simulink model "exintercol"  (R2018a)
settings: Solver=FixedStepDiscrete  StartTime=0.0  StopTime=500  RelTol=1e-3  EnableMultiTasking=on
values from neighbouring files (symbols this model uses):
  lt = 3    [examplesupplychainCIO.m]
undefined symbols (not defined in the file or in its folder): magnitude, norminv
settings Model: Creator=Juan Ramón Trapero  LastModifiedBy=azken
settings DataIOCC: LimitDataPoints=on  SaveFormat=Array  SignalLoggingSaveFormat=ModelDataLogs
settings OptimizationCC: ExpressionDepthLimit=2147483647  InitFltsAndDblsToZero=on  LifeSpan=inf
settings DebuggingCC: UnderspecifiedInitializationDetection=Classic  MergeDetectMultiDrivingBlocksExec=none  SolverPrmCheckMsg=warning  FcnCallInpInsideContextMsg=warning  StateNameClashWarn=warning  SFUnexpectedBacktrackingDiag=warning  SFNoUnconditionalDefaultTransitionDiag=warning  SFExecutionAtInitializationDiag=none
settings HardwareCC: ProdBitPerPointer=32  ProdBitPerSizeT=32  ProdBitPerPtrDiffT=32  ProdLargestAtomicFloat=None  ProdIntDivRoundTo=Undefined  ProdEndianess=Unspecified  ProdWordSize=32  ProdHWDeviceType=32-bit Generic
settings ModelReferenceCC: PropagateSignalLabelsOutOfModel=off
settings CodeAppCC: StateflowObjectComments=on
settings GRTTargetCC: TargetLangStandard=C89/C90 (ANSI)  GeneratePreprocessorConditionals=Disable all  CombineOutputUpdateFcns=off  GRTInterface=on
settings ConfigComp: CovMetricSettings=dw  CovHtmlReporting=on  CovSaveCumulativeToWorkspaceVar=on  CovSaveSingleToWorkspaceVar=on  CovExternalEMLEnable=off

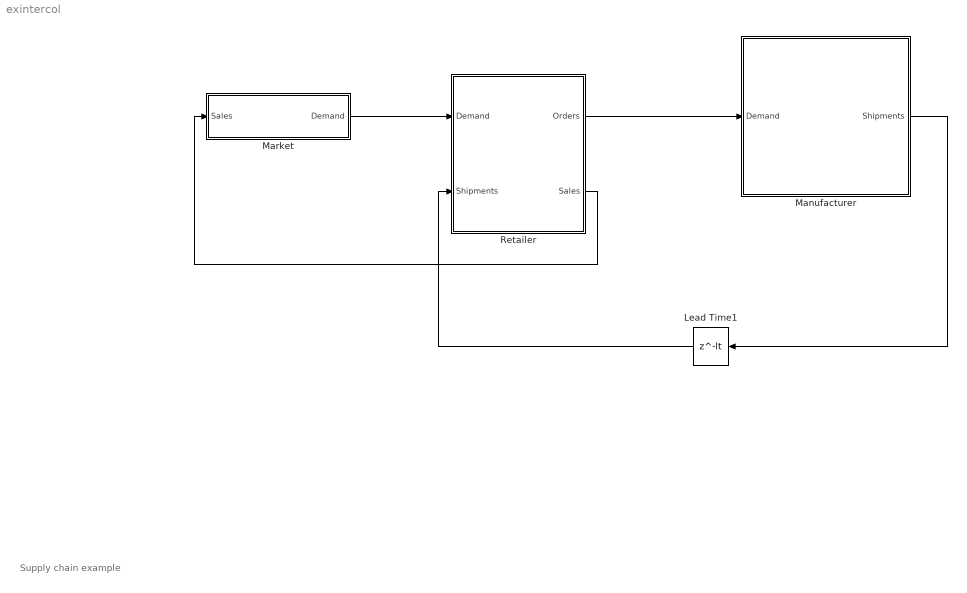
== system exintercol ==
  note: Supply chain example
  Lead Time1 : Delay  DelayLength=lt  InputProcessing=Inherited
  Manufacturer : Subsystem  AncestorBlock=SCMSv2016a/Supply Chain Members/Manufacturer
  Market : Subsystem  AncestorBlock=SCMSv2016a/Supply Chain Members/Market
  Retailer : Subsystem  AncestorBlock=SCMSv2016a/Supply Chain Members/Retailer
  wires:
  Manufacturer/1(Shipments) -> Lead Time1/1
  Lead Time1/1 -> Retailer/2(Shipments)
  Market/1(Demand) -> Retailer/1(Demand)
  Retailer/2(Sales) -> Market/1(Sales)
  Retailer/1(Orders) -> Manufacturer/1(Demand)

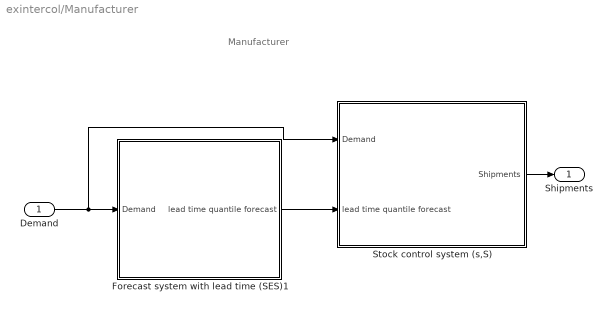
== system exintercol/Manufacturer ==
  note: Manufacturer
  Demand : Inport
  Forecast system with lead time (SES)1 : Subsystem  AncestorBlock=SCMSv2016a/Forecasting policies/Forecast system with lead time (SES)  mask{alpha1=0.1, ini1=100, alpha2=0.01, ini2=15, k=norminv(0.95,0,1);, lt=3}
      mask prompts: alpha1 "SES constant (alpha1)"; alpha2 "SES constant (alpha2)"; k "safety factor (k)"; lt "lead time"
      mask help:
      | This block computes the lead time quantile forecast of the demand. Please, see the block help for more details about block parameters.
      | Usually the output of this block is fed to stock control blocks to determine the reorder point.
      mask Help:
      | Input: Demand
      | Output:
      |    Lead time quantile forecast.
      | Parameters:
      |    alpha1: exponential smoothing constant used to compute mean forecast.
      |    ini1: initial forecast used by exponential smoothing regarding mean forecast.
      |    alpha2: exponential smoothing constant used to compute variance forecast.
      |    ini2: initial forecast used by exponential smoothing regarding variance forecast.
      |    k: safety factor that depends on the cycle service level (quantile).
      |    lead time.
  Stock control system (s,S) : Subsystem  mask{S=2000, Tp=3}
  Shipments : Outport
  wires:
  Demand/1 -> Stock control system (s,S)/1(Demand), Forecast system with lead time (SES)1/1(Demand)
  Forecast system with lead time (SES)1/1(lead time quantile forecast) -> Stock control system (s,S)/2(lead time quantile forecast)
  Stock control system (s,S)/1(Shipments) -> Shipments/1

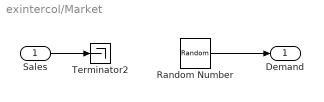
== system exintercol/Market ==
  Sales : Inport
  Random Number : RandomNumber  Mean=100  Variance=20  SampleTime=1
  Terminator2 : Terminator
  Demand : Outport
  wires:
  Sales/1 -> Terminator2/1
  Random Number/1 -> Demand/1

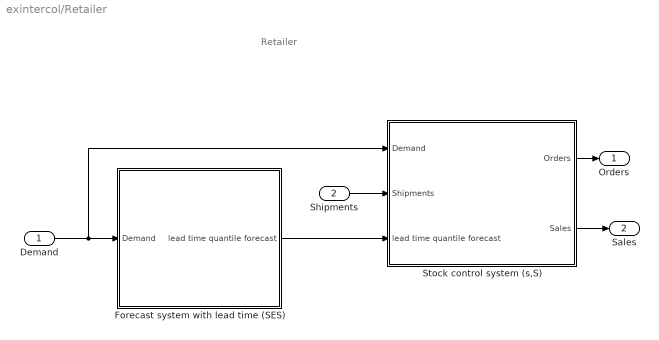
== system exintercol/Retailer ==
  note: Retailer
  Demand : Inport
  Shipments : Inport  Port=2
  Forecast system with lead time (SES) : Subsystem  AncestorBlock=SCMSv2016a/Forecasting policies/Forecast system with lead time (SES)  mask{alpha1=0.1, ini1=100, alpha2=0.010, ini2=15, k=norminv(0.95,0,1), lt=3}
      mask prompts: alpha1 "SES constant (alpha1)"; alpha2 "SES constant (alpha2)"; k "safety factor (k)"; lt "lead time"
      mask help:
      | This block computes the lead time quantile forecast of the demand. Please, see the block help for more details about block parameters.
      | Usually the output of this block is fed to stock control blocks to determine the reorder point.
      mask Help:
      | Input: Demand
      | Output:
      |    Lead time quantile forecast.
      | Parameters:
      |    alpha1: exponential smoothing constant used to compute mean forecast.
      |    ini1: initial forecast used by exponential smoothing regarding mean forecast.
      |    alpha2: exponential smoothing constant used to compute variance forecast.
      |    ini2: initial forecast used by exponential smoothing regarding variance forecast.
      |    k: safety factor that depends on the cycle service level (quantile).
      |    lead time.
  Stock control system (s,S) : Subsystem  mask{S=1000}
  Orders : Outport
  Sales : Outport  Port=2
  wires:
  Demand/1 -> Stock control system (s,S)/1(Demand), Forecast system with lead time (SES)/1(Demand)
  Forecast system with lead time (SES)/1(lead time quantile forecast) -> Stock control system (s,S)/3(lead time quantile forecast)
  Stock control system (s,S)/2(Sales) -> Sales/1
  Stock control system (s,S)/1(Orders) -> Orders/1
  Shipments/1 -> Stock control system (s,S)/2(Shipments)

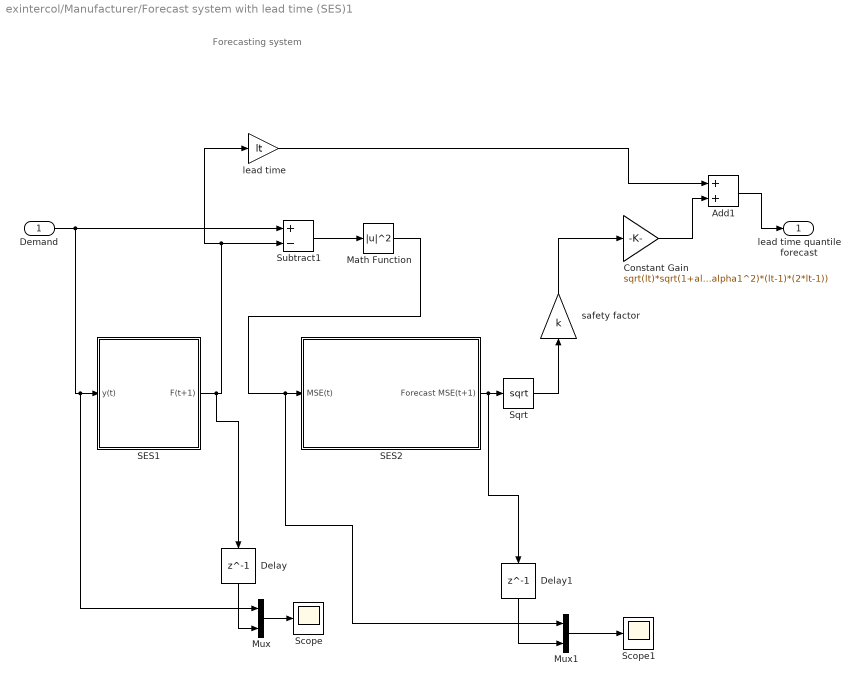
== system exintercol/Manufacturer/Forecast system with lead time (SES)1 ==
  note: Forecasting system
  Demand : Inport
  Add1 : Sum
  Constant Gain : Gain  Gain=sqrt(lt)*sqrt(1+alpha1*(lt-1)+1/6*(alpha1^2)*(lt-1)*(2*lt-1))
  Delay : Delay  DelayLength=1  InitialCondition=ini1
  Delay1 : Delay  DelayLength=1  InitialCondition=ini2
  Math Function : Math  Operator=magnitude^2  SaturateOnIntegerOverflow=on
  Mux : Mux  Inputs=2
  Mux1 : Mux  Inputs=2
  SES1 : Subsystem
  SES2 : Subsystem
  Scope : Scope
  Scope1 : Scope
  Sqrt : Sqrt  SaturateOnIntegerOverflow=on
  Subtract1 : Sum  Inputs=+-
  lead time : Gain  Gain=lt
  safety factor : Gain  Gain=k
  lead time quantile forecast : Outport
  wires:
  SES1/1(F(t+1)) -> Delay/1, lead time/1, Subtract1/2
  Subtract1/1 -> Math Function/1
  Sqrt/1 -> safety factor/1
  SES2/1(Forecast MSE(t+1)) -> Delay1/1, Sqrt/1
  lead time/1 -> Add1/1
  safety factor/1 -> Constant Gain/1
  Constant Gain/1 -> Add1/2
  Add1/1 -> lead time quantile forecast/1
  Math Function/1 -> Mux1/1, SES2/1(MSE(t))
  Demand/1 -> Subtract1/1, Mux/1, SES1/1(y(t))
  Mux1/1 -> Scope1/1
  Mux/1 -> Scope/1
  Delay/1 -> Mux/2
  Delay1/1 -> Mux1/2

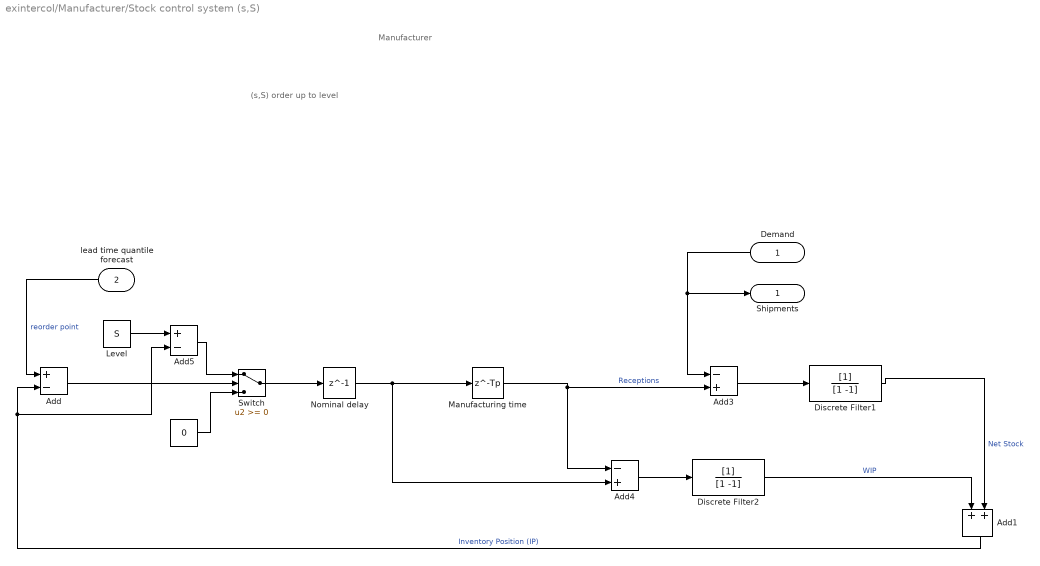
== system exintercol/Manufacturer/Stock control system (s,S) ==
  note: (s,S) order up to level
  note: Manufacturer
  Demand : Inport
  lead time quantile forecast : Inport  Port=2
  " " : Constant  Value=0
  Add : Sum  Inputs=+-
  Add1 : Sum
  Add3 : Sum  Inputs=-+
  Add4 : Sum  Inputs=-+
  Add5 : Sum  Inputs=+-
  Discrete Filter1 : DiscreteFilter  Denominator=[1 -1]  SampleTime=1
  Discrete Filter2 : DiscreteFilter  Denominator=[1 -1]  SampleTime=1
  Level : Constant  Value=S
  Manufacturing time : Delay  DelayLength=Tp  InputProcessing=Inherited
  Nominal delay : Delay  DelayLength=1  InputProcessing=Inherited
  Switch : Switch
  Shipments : Outport
  wires:
  lead time quantile forecast/1 -> Add/1  "reorder point"
  " "/1 -> Switch/3
  Add4/1 -> Discrete Filter2/1
  Demand/1 -> Shipments/1, Add3/1
  Add3/1 -> Discrete Filter1/1
  Level/1 -> Add5/1
  Add/1 -> Switch/2
  Nominal delay/1 -> Add4/2, Manufacturing time/1
  Discrete Filter1/1 -> Add1/2  "Net Stock"
  Add1/1 -> Add5/2, Add/2  "Inventory Position (IP)"
  Add5/1 -> Switch/1
  Manufacturing time/1 -> Add4/1, Add3/2  "Receptions"
  Discrete Filter2/1 -> Add1/1  "WIP"
  Switch/1 -> Nominal delay/1

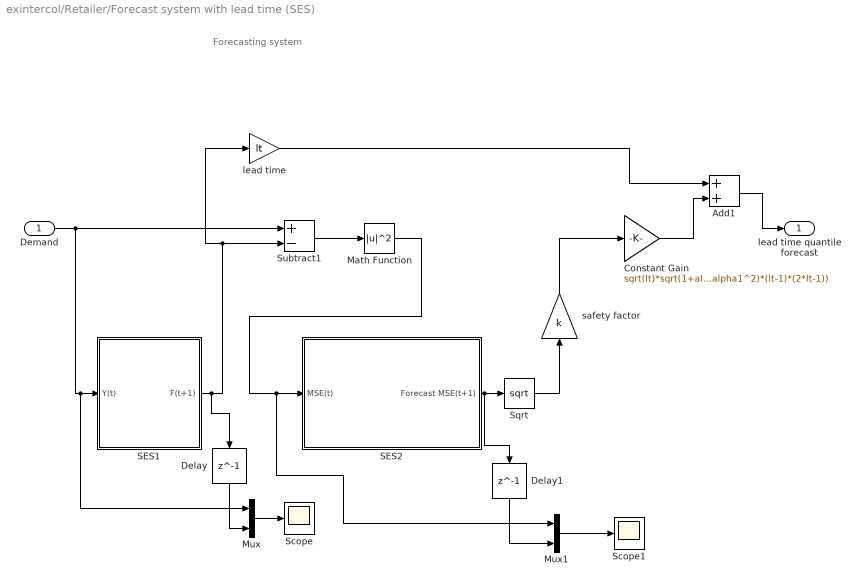
== system exintercol/Retailer/Forecast system with lead time (SES) ==
  note: Forecasting system
  Demand : Inport
  Add1 : Sum
  Constant Gain : Gain  Gain=sqrt(lt)*sqrt(1+alpha1*(lt-1)+1/6*(alpha1^2)*(lt-1)*(2*lt-1))
  Delay : Delay  DelayLength=1  InitialCondition=ini1
  Delay1 : Delay  DelayLength=1  InitialCondition=ini2
  Math Function : Math  Operator=magnitude^2  SaturateOnIntegerOverflow=on
  Mux : Mux  Inputs=2
  Mux1 : Mux  Inputs=2
  SES1 : Subsystem
  SES2 : Subsystem
  Scope : Scope
  Scope1 : Scope
  Sqrt : Sqrt  SaturateOnIntegerOverflow=on
  Subtract1 : Sum  Inputs=+-
  lead time : Gain  Gain=lt
  safety factor : Gain  Gain=k
  lead time quantile forecast : Outport
  wires:
  Add1/1 -> lead time quantile forecast/1
  Constant Gain/1 -> Add1/2
  safety factor/1 -> Constant Gain/1
  lead time/1 -> Add1/1
  SES2/1(Forecast MSE(t+1)) -> Delay1/1, Sqrt/1
  Sqrt/1 -> safety factor/1
  Subtract1/1 -> Math Function/1
  Math Function/1 -> Mux1/1, SES2/1(MSE(t))
  SES1/1(F(t+1)) -> Delay/1, Subtract1/2, lead time/1
  Demand/1 -> Mux/1, SES1/1(Y(t)), Subtract1/1
  Mux1/1 -> Scope1/1
  Mux/1 -> Scope/1
  Delay/1 -> Mux/2
  Delay1/1 -> Mux1/2

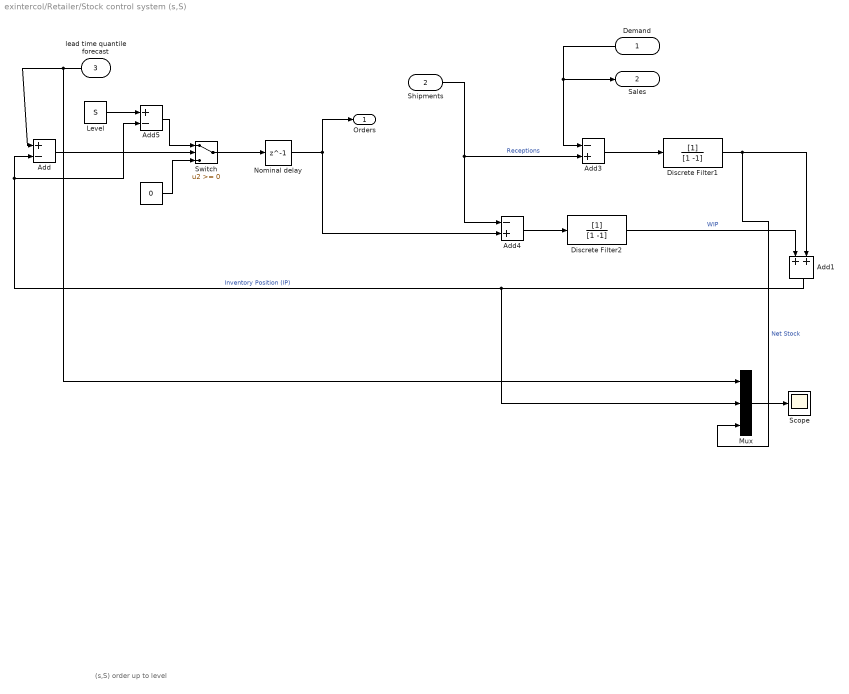
== system exintercol/Retailer/Stock control system (s,S) ==
  note: (s,S) order up to level
  Demand : Inport
  Shipments : Inport  Port=2
  lead time quantile forecast : Inport  Port=3
  " " : Constant  Value=0
  Add : Sum  Inputs=+-
  Add1 : Sum
  Add3 : Sum  Inputs=-+
  Add4 : Sum  Inputs=-+
  Add5 : Sum  Inputs=+-
  Discrete Filter1 : DiscreteFilter  Denominator=[1 -1]  SampleTime=1
  Discrete Filter2 : DiscreteFilter  Denominator=[1 -1]  SampleTime=1
  Level : Constant  Value=S
  Mux : Mux  Inputs=3
  Nominal delay : Delay  DelayLength=1  InputProcessing=Inherited
  Scope : Scope
  Switch : Switch
  Orders : Outport
  Sales : Outport  Port=2
  wires:
  lead time quantile forecast/1 -> Mux/1, Add/1
  " "/1 -> Switch/3
  Add4/1 -> Discrete Filter2/1
  Demand/1 -> Sales/1, Add3/1
  Add3/1 -> Discrete Filter1/1
  Level/1 -> Add5/1
  Add/1 -> Switch/2
  Nominal delay/1 -> Orders/1, Add4/2
  Discrete Filter1/1 -> Mux/3, Add1/2  "Net Stock"
  Add1/1 -> Mux/2, Add5/2, Add/2  "Inventory Position (IP)"
  Add5/1 -> Switch/1
  Shipments/1 -> Add4/1, Add3/2  "Receptions"
  Discrete Filter2/1 -> Add1/1  "WIP"
  Switch/1 -> Nominal delay/1
  Mux/1 -> Scope/1

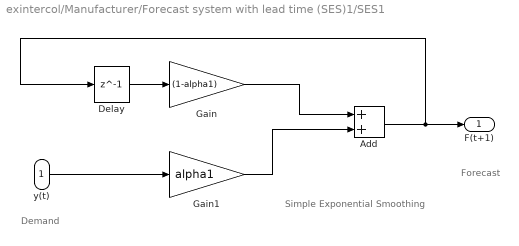
== system exintercol/Manufacturer/Forecast system with lead time (SES)1/SES1 ==
  note: Simple Exponential Smoothing
  note: Forecast
  note: Demand
  y(t) : Inport
  Add : Sum
  Delay : Delay  DelayLength=1  InitialCondition=ini1
  Gain : Gain  Gain=(1-alpha1)
  Gain1 : Gain  Gain=alpha1
  F(t+1) : Outport
  wires:
  Gain/1 -> Add/1
  Delay/1 -> Gain/1
  Gain1/1 -> Add/2
  y(t)/1 -> Gain1/1
  Add/1 -> F(t+1)/1, Delay/1

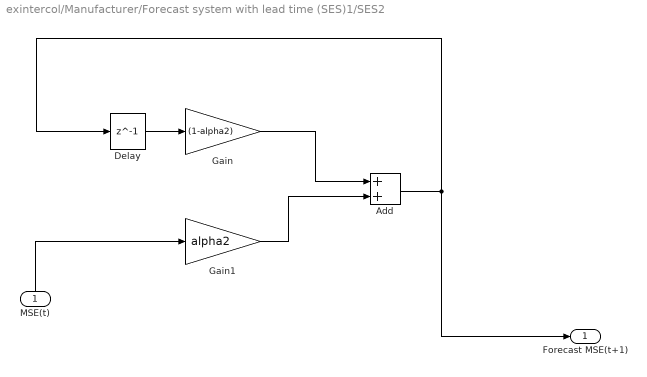
== system exintercol/Manufacturer/Forecast system with lead time (SES)1/SES2 ==
  MSE(t) : Inport
  Add : Sum
  Delay : Delay  DelayLength=1  InitialCondition=ini2
  Gain : Gain  Gain=(1-alpha2)
  Gain1 : Gain  Gain=alpha2
  Forecast MSE(t+1) : Outport
  wires:
  Gain/1 -> Add/1
  Delay/1 -> Gain/1
  Gain1/1 -> Add/2
  MSE(t)/1 -> Gain1/1
  Add/1 -> Forecast MSE(t+1)/1, Delay/1

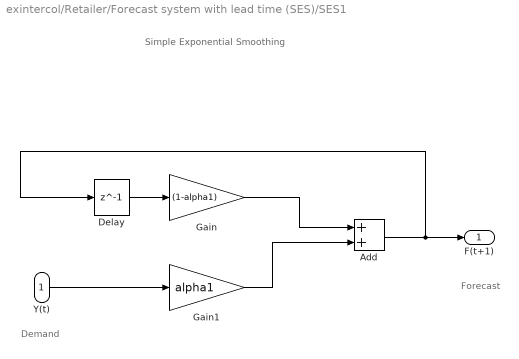
== system exintercol/Retailer/Forecast system with lead time (SES)/SES1 ==
  note: Demand
  note: Forecast
  note: Simple Exponential Smoothing
  Y(t) : Inport
  Add : Sum
  Delay : Delay  DelayLength=1  InitialCondition=ini1
  Gain : Gain  Gain=(1-alpha1)
  Gain1 : Gain  Gain=alpha1
  F(t+1) : Outport
  wires:
  Add/1 -> Delay/1, F(t+1)/1
  Y(t)/1 -> Gain1/1
  Gain1/1 -> Add/2
  Delay/1 -> Gain/1
  Gain/1 -> Add/1

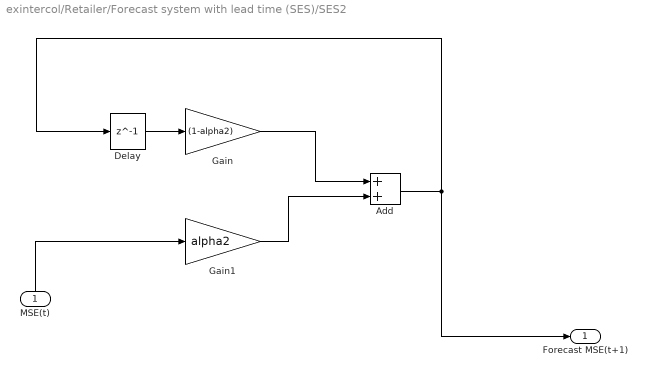
== system exintercol/Retailer/Forecast system with lead time (SES)/SES2 ==
  MSE(t) : Inport
  Add : Sum
  Delay : Delay  DelayLength=1  InitialCondition=ini2
  Gain : Gain  Gain=(1-alpha2)
  Gain1 : Gain  Gain=alpha2
  Forecast MSE(t+1) : Outport
  wires:
  Add/1 -> Delay/1, Forecast MSE(t+1)/1
  MSE(t)/1 -> Gain1/1
  Gain1/1 -> Add/2
  Delay/1 -> Gain/1
  Gain/1 -> Add/1
